simulink model "EL7221_HexaPKM"  (Simulink 9.2)
settings: Solver=FixedStepDiscrete  StartTime=0.0  StopTime=inf  FixedStep=param.t_sample  RelTol=1e-3
InitFcn:
  | %mdl_name = mdlName_simulink;
  | %try
  | %resetTrajBlocks(mdl_name, 'Zielposition/Trajektorie', param.len_traj_max);
  | %catch
  | %resetTrajBlocks(mdl_name, 'Zielposition/Trajektorie', 60000);
  | %end
  | 
  | set_param(bdroot,'ExtModeMexArgs', mex_file_args)
undefined symbols (not defined in the file or in its folder): param_drive
undefined symbols (not defined in the file): drive_idx, EL7221_HexaPKM
libraries: simulink x3
PreSaveFcn:
  | mdl_name = mdlName_simulink;
  | try
  | resetTrajBlocks(mdl_name, 'Zielposition/Trajektorie', param.len_traj_max);
  | catch
  | resetTrajBlocks(mdl_name, 'Zielposition/Trajektorie', 60000);
  | end
settings Model: Creator=schappler  LastModifiedBy=pkr_devpc  SimulationMode=external  EnablePacing=on  ExtModeTrigDuration=10000  ExtModeArchiveMode=auto  ExtModeArchiveFileName=measurement_data  ExtModeArchiveDirName=./results  ExtModeLogAll=off
settings SolverCC: MinimalZcImpactIntegration=on
settings DataIOCC: LimitDataPoints=off  SaveFormat=Dataset  SignalLoggingSaveFormat=Dataset  SaveOutput=off  SignalLogging=off  SaveTime=off
settings OptimizationCC: BufferReuse=off  GlobalBufferReuse=off  ExpressionFolding=off  LocalBlockOutputs=off  LifeSpan=auto  OptimizeDataStoreBuffers=off  BusAssignmentInplaceUpdate=off
settings DebuggingCC: ReadBeforeWriteMsg=DisableAll  WriteAfterWriteMsg=DisableAll  WriteAfterReadMsg=DisableAll  UnderspecifiedInitializationDetection=Simplified  MergeDetectMultiDrivingBlocksExec=error  MultiTaskDSMMsg=none  FcnCallInpInsideContextMsg=error  StateNameClashWarn=none  SFUnexpectedBacktrackingDiag=error  SFNoUnconditionalDefaultTransitionDiag=error  SFExecutionAtInitializationDiag=warning
settings HardwareCC: ProdBitPerPointer=64  ProdBitPerSizeT=64  ProdBitPerPtrDiffT=64  ProdLargestAtomicFloat=Float  ProdIntDivRoundTo=Zero  ProdEndianess=LittleEndian  ProdWordSize=64  ProdHWDeviceType=Intel->x86-64 (Windows64)
settings ModelReferenceCC: UpdateModelReferenceTargets=IfOutOfDate  PropagateSignalLabelsOutOfModel=on
settings SFSimCC: SFSimEcho=off  SimUseLocalCustomCode=on
settings RTWCC: SystemTargetFile=etherlab.tlc  TemplateMakefile=etherlab_hrt.tmf  Description=EtherLab PREEMT_RT Real-Time Target  GenerateReport=on  RTWUseLocalCustomCode=on  LaunchReport=on
settings CodeAppCC: StateflowObjectComments=off
settings STFCustomTargetCC: TargetLangStandard=C99 (ISO)  SystemTargetFile=etherlab.tlc
settings GRTTargetCC: TargetLangStandard=C99 (ISO)  ParMdlRefBuildCompliant=off  CompOptLevelCompliant=off  ConcurrentExecutionCompliant=off  GeneratePreprocessorConditionals=Use local settings  MatFileLogging=off  CPPClassGenCompliant=off  UseToolchainInfoCompliant=off  ExtMode=on  ExtModeStaticAlloc=on  ExtModeStaticAllocSize=80000000  ExtModeMexArgs='10.144.130.77' 0 17725  RTWCAPISignals=on  RTWCAPIParams=on
settings CustomProperty: DataType=int32  Value=2
settings ConfigComp: CovMetricSettings=dwe  CovHtmlReporting=off  CovSaveCumulativeToWorkspaceVar=off  CovSaveSingleToWorkspaceVar=off  CovExternalEMLEnable=on

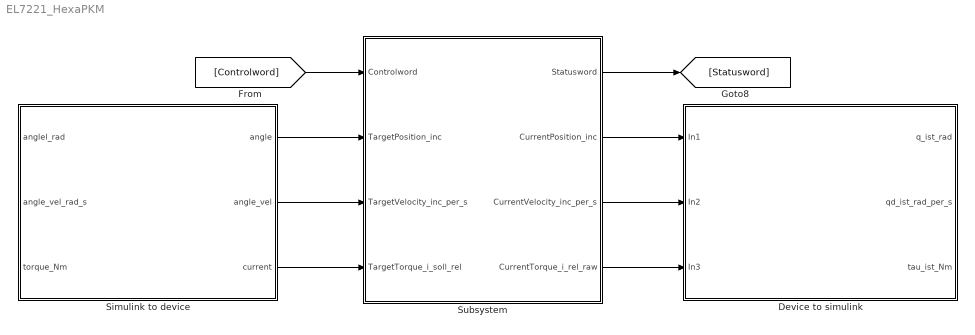
== system EL7221_HexaPKM ==
  Device to simulink : Subsystem
  Simulink to device : Subsystem
  Subsystem : Subsystem
  wires:
  Subsystem/3(CurrentVelocity_inc_per_s) -> Device to simulink/2(In2)
  Simulink to device/3(current) -> Subsystem/4(TargetTorque_i_soll_rel)
  Subsystem/4(CurrentTorque_i_rel_raw) -> Device to simulink/3(In3)
  Subsystem/2(CurrentPosition_inc) -> Device to simulink/1(In1)
  Subsystem/1(Statusword) -> [Statusword]
  Simulink to device/1(angle) -> Subsystem/2(TargetPosition_inc)
  Simulink to device/2(angle_vel) -> Subsystem/3(TargetVelocity_inc_per_s)
  [Controlword] -> Subsystem/1(Controlword)

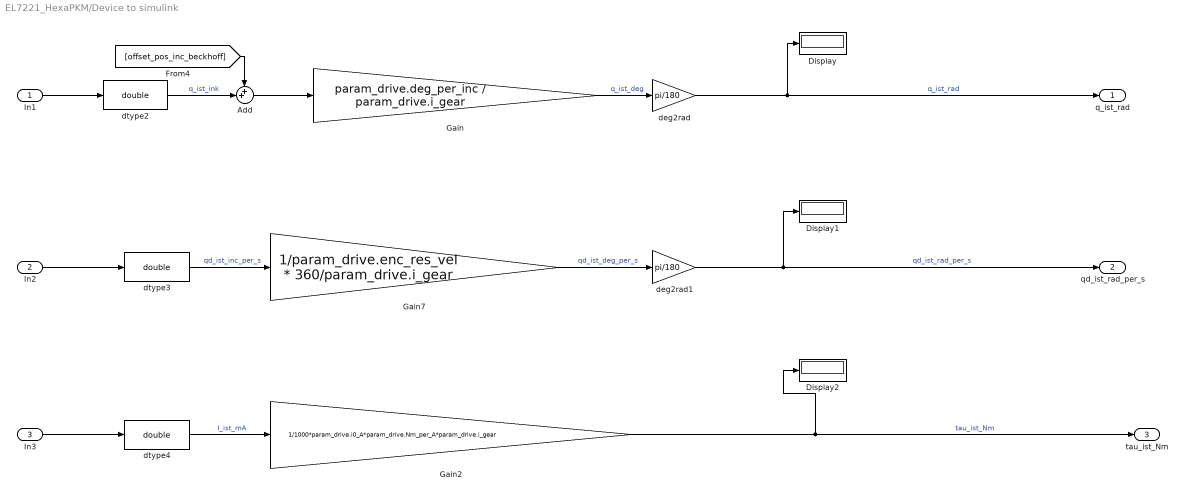
== system EL7221_HexaPKM/Device to simulink ==
  In1 : Inport
  In2 : Inport  Port=2
  In3 : Inport  Port=3
  Add : Sum  Inputs=++|
  Display : Display
  Display1 : Display
  Display2 : Display
  Gain : Gain  Gain=param_drive.deg_per_inc / param_drive.i_gear
  Gain2 : Gain  Gain=1/1000*param_drive.i0_A*param_drive.Nm_per_A*param_drive.i_gear
  Gain7 : Gain  Gain=1/param_drive.enc_res_vel * 360/param_drive.i_gear
  deg2rad : Gain  Gain=pi/180
  deg2rad1 : Gain  Gain=pi/180
  dtype2 : DataTypeConversion  OutDataTypeStr=double
  dtype3 : DataTypeConversion  OutDataTypeStr=double
  dtype4 : DataTypeConversion  OutDataTypeStr=double
  q_ist_rad : Outport
  qd_ist_rad_per_s : Outport  Port=2
  tau_ist_Nm : Outport  Port=3
  wires:
  dtype2/1 -> Add/2  "q_ist_ink"
  [offset_pos_inc_beckhoff] -> Add/1
  In3/1 -> dtype4/1
  Gain2/1 -> tau_ist_Nm/1, Display2/1  "tau_ist_Nm"
  deg2rad1/1 -> qd_ist_rad_per_s/1, Display1/1  "qd_ist_rad_per_s"
  Gain7/1 -> deg2rad1/1  "qd_ist_deg_per_s"
  deg2rad/1 -> q_ist_rad/1, Display/1  "q_ist_rad"
  Gain/1 -> deg2rad/1  "q_ist_deg"
  Add/1 -> Gain/1
  dtype3/1 -> Gain7/1  "qd_ist_inc_per_s"
  In2/1 -> dtype3/1
  In1/1 -> dtype2/1
  dtype4/1 -> Gain2/1  "I_ist_mA"

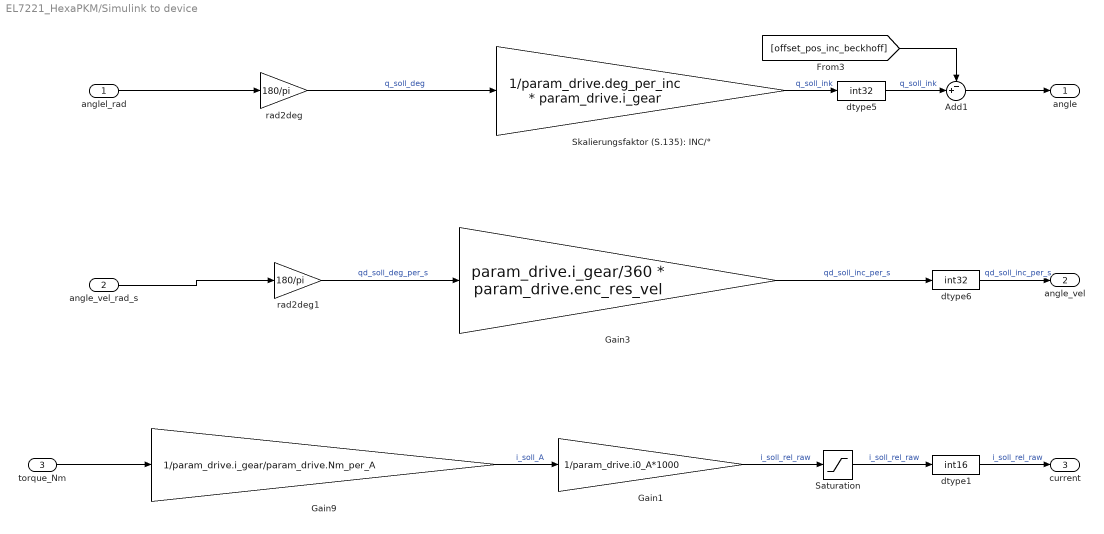
== system EL7221_HexaPKM/Simulink to device ==
  anglel_rad : Inport
  angle_vel_rad_s : Inport  Port=2
  torque_Nm : Inport  Port=3
  Add1 : Sum  Inputs=-+|
  Gain1 : Gain  Gain=1/param_drive.i0_A*1000
  Gain3 : Gain  Gain=param_drive.i_gear/360 * param_drive.enc_res_vel
  Gain9 : Gain  Gain=1/param_drive.i_gear/param_drive.Nm_per_A
  Saturation : Saturate  UpperLimit=param_drive.i_lim_rel(2)  LowerLimit=param_drive.i_lim_rel(1)
  Skalierungsfaktor (S.135): INC/° : Gain  Gain=1/param_drive.deg_per_inc * param_drive.i_gear
  dtype1 : DataTypeConversion  OutDataTypeStr=int16
  dtype5 : DataTypeConversion  OutDataTypeStr=int32
  dtype6 : DataTypeConversion  OutDataTypeStr=int32
  rad2deg : Gain  Gain=180/pi
  rad2deg1 : Gain  Gain=180/pi
  angle : Outport
  angle_vel : Outport  Port=2
  current : Outport  Port=3
  wires:
  Gain3/1 -> dtype6/1  "qd_soll_inc_per_s"
  rad2deg1/1 -> Gain3/1  "qd_soll_deg_per_s"
  Add1/1 -> angle/1
  Saturation/1 -> dtype1/1  "i_soll_rel_raw"
  Gain1/1 -> Saturation/1  "i_soll_rel_raw"
  dtype1/1 -> current/1  "i_soll_rel_raw"
  [offset_pos_inc_beckhoff] -> Add1/1
  angle_vel_rad_s/1 -> rad2deg1/1
  dtype5/1 -> Add1/2  "q_soll_ink"
  torque_Nm/1 -> Gain9/1
  Gain9/1 -> Gain1/1  "i_soll_A"
  anglel_rad/1 -> rad2deg/1
  dtype6/1 -> angle_vel/1  "qd_soll_inc_per_s"
  rad2deg/1 -> Skalierungsfaktor (S.135): INC/°/1  "q_soll_deg"
  Skalierungsfaktor (S.135): INC/°/1 -> dtype5/1  "q_soll_ink"

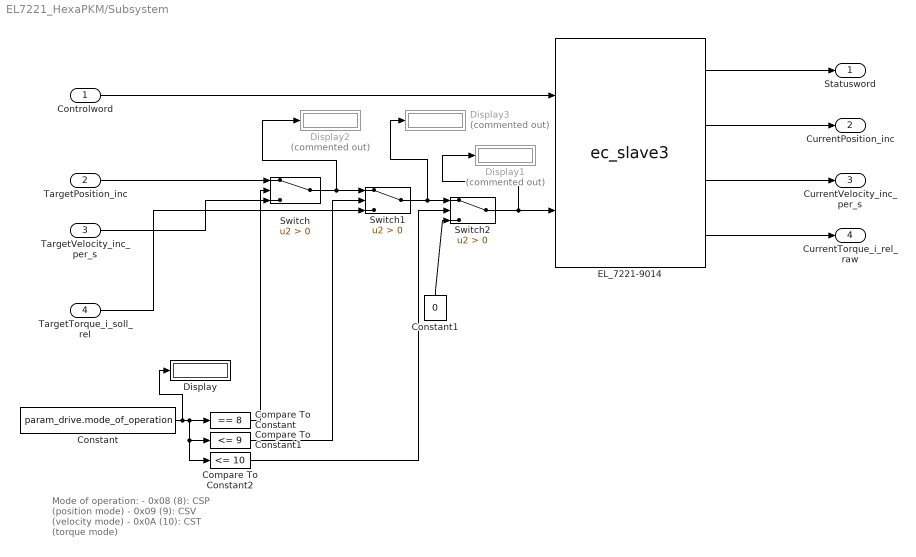
== system EL7221_HexaPKM/Subsystem ==
  note: Mode of operation:
      | - 0x08 (8): CSP (position mode)
      | - 0x09 (9): CSV (velocity mode)
      | - 0x0A (10): CST (torque mode)
  Controlword : Inport
  TargetPosition_inc : Inport  Port=2
  TargetVelocity_inc_per_s : Inport  Port=3
  TargetTorque_i_soll_rel : Inport  Port=4
  Compare To Constant : simulink/Logic and Bit Operations/Compare To Constant  relop===  const=8  OutDataTypeStr=boolean
  Compare To Constant1 : simulink/Logic and Bit Operations/Compare To Constant  relop=<=  const=9  OutDataTypeStr=boolean
  Compare To Constant2 : simulink/Logic and Bit Operations/Compare To Constant  relop=<=  const=10  OutDataTypeStr=boolean
  Constant : Constant  Value=param_drive.mode_of_operation  SampleTime=-1
  Constant1 : Constant  Value=0  SampleTime=-1
  Display : Display
  Display1 : Display  Commented=on
  Display2 : Display  Commented=on
  Display3 : Display  Commented=on
  "EL_7221-9014 " : S-Function  AncestorBlock=etherlab_lib/EtherCAT/Generic_0  FunctionName=ec_slave3  Parameters=Address,rv.SlaveConfig,rv.PortConfig,debug,tsample,param  SFunctionModules='ecrt_support'  SFunctionDeploymentMode=off  EnableBusSupport=off  mask(Generic EtherCAT Slave){master=0, index=drive_idx, rv=EL7221_HexaPKM(param_drive.mode_of_operation), param=[], tsample=0.001, debug=0}
      mask prompts: index "Slave Index"; rv "EtherCAT Slave Configuration struct. (SlaveConfig, PortConfig)"; param "Block Parameters"; tsample "Sample Time"
      mask help:
      | The generic EtherCAT Slave is used to create any slave not contained
      | in this library. A mask input variable, <b>EtherCAT Slave Configuration</b>,
      | has to be set up by the user. This configures the slave.
      mask init:
      | Address = EtherCATSlave.formatAddress(master,index,tsample);
      | 
      | if ~isfield(rv,'PortConfig') || isempty(rv)
      |    rv.PortConfig = [];
      | end
      | 
      | if ~isfield(rv,'SlaveConfig') || isempty(rv)
      |    rv.SlaveConfig = [];
      | end
      | 
      | if ~isfield(rv.SlaveConfig,'description') || isempty(rv)
      |    slave_name = 'unknown';
      | else
      |    slave_name = rv.SlaveConfig.description;
      | end
      mask Help: web(etherlab_help_path('generic.html'), '-helpbrowser');
      mask Display:
      | fprintf('Generic Slave\n%s \n%i Idx:%s', ...
      |     slave_name, master, mat2str(index))
  Switch : Switch  Criteria=u2 > Threshold
  Switch1 : Switch  Criteria=u2 > Threshold
  Switch2 : Switch  Criteria=u2 > Threshold
  Statusword : Outport
  CurrentPosition_inc : Outport  Port=2
  CurrentVelocity_inc_per_s : Outport  Port=3
  CurrentTorque_i_rel_raw : Outport  Port=4
  wires:
  TargetPosition_inc/1 -> Switch/1
  Compare To Constant2/1 -> Switch2/2
  Compare To Constant1/1 -> Switch1/2
  Controlword/1 -> "EL_7221-9014 "/1
  Constant/1 -> Compare To Constant/1, Compare To Constant1/1, Compare To Constant2/1, Display/1
  "EL_7221-9014 "/2 -> CurrentPosition_inc/1
  "EL_7221-9014 "/4 -> CurrentTorque_i_rel_raw/1
  Switch2/1 -> Display1/1, "EL_7221-9014 "/2
  Switch1/1 -> Switch2/1, Display3/1
  TargetVelocity_inc_per_s/1 -> Switch/3
  "EL_7221-9014 "/1 -> Statusword/1
  Switch/1 -> Switch1/1, Display2/1
  TargetTorque_i_soll_rel/1 -> Switch1/3
  Compare To Constant/1 -> Switch/2
  "EL_7221-9014 "/3 -> CurrentVelocity_inc_per_s/1
  Constant1/1 -> Switch2/3
